simulink model "orbit_propagator_matlab2023b"  (R2023b)
settings: Solver=FixedStepAuto  StartTime=0.0  StopTime=207944  FixedStep=sim_step_size  RelTol=1e-6  AbsTol=1e-7
model workspace (MAT data in the model file):
  current_year = 2025
  year = 2013
values from neighbouring files (symbols this model uses):
  alpha_acc = sqrt(0.7)    [HSat_op_setup_merged_maria.m]    (also in init_orbit_analysis_with_drag_loss.m)
  aph = 200*ones(1,7)    [init_orbit_analysis_with_drag_loss.m]
  COM = [0, 0, 0.25+0.3]    [init_orbit_analysis_with_drag_loss.m]
  ext_ENV_muEarth = 3.986005e14    (= 398600500000000)    [GEO_insertion_setup.m]    (also in HSat_op_setup.m; HSat_op_setup_merged_maria.m; init_orbit_analysis_with_drag_loss.m)
  F107 = 300    [init_orbit_analysis_with_drag_loss.m]
  P_solar = 4.56e-6    (= 4.56e-06)    [HSat_op_setup_merged_maria.m]    (also in init_orbit_analysis_with_drag_loss.m)
  perigee_vector_eci = [0, 1, 0]    [init_orbit_analysis_with_drag_loss.m]
  sim_SC_init_MoI_EOR_wet = [ ... (first row only)    [HSat_op_setup.m]    (also in HSat_op_setup_merged_maria.m; init_orbit_analysis_with_drag_loss.m)
  sim_step_size = 10    [init_orbit_analysis_with_drag_loss.m]
  sun_pointing = 1    [init_orbit_analysis_with_drag_loss.m]
  sun_pointing_SA = 0    [HSat_op_setup_merged_maria.m]    (also in init_orbit_analysis_with_drag_loss.m)
  theta = deg2rad(0)    [init_orbit_analysis_with_drag_loss.m]
undefined symbols (not defined in the file or in its folder): attitude, sun_vector_oc
libraries: aerolibutil x37, matrix_library x37, Toolbox x10, sharedtransform x10, aerolibatmos2 x1, simulink x1, simulink_extras x1
(part 3 of 3)

== system orbit_propagator_matlab2023b/Disturbing torques/sc area projected to v // aero drag torque // srp torque/Switch Case Action Subsystem/sun pointing solar arrays/Nomalize_noDivideByZero1 ==
  e : Inport
  2-norm : Subsystem
      mask Display: disp('||u||')
  Product : Product  Inputs=*/  InputSameDT=on  RndMeth=Zero  SaturateOnIntegerOverflow=on  OutDataTypeStr=Inherit: Same as first input
  Switch : Switch  Criteria=u2 > Threshold  SaturateOnIntegerOverflow=off  InputSameDT=off
  zero : Constant  Value=0
  ehat : Outport
  wires:
  e/1 -> 2-norm/1(In1), Product/1
  2-norm/1(Out1) -> Switch/2, Product/2
  Switch/1 -> ehat/1
  Product/1 -> Switch/1
  zero/1 -> Switch/3

== system orbit_propagator_matlab2023b/Disturbing torques/sc area projected to v // aero drag torque // srp torque/z -1/Nomalize_noDivideByZero/2-norm ==
  In1 : Inport
  Math Function : Math  Operator=sqrt  SignedPower=on
  Product1 : Product  InputSameDT=on  RndMeth=Zero  SaturateOnIntegerOverflow=on  OutDataTypeStr=Inherit: Same as first input
  Sum : Sum  Inputs=+  InputSameDT=on  SaturateOnIntegerOverflow=on  OutDataTypeStr=Inherit: Same as first input
  Out1 : Outport
  wires:
  In1/1 -> Product1/1, Product1/2
  Product1/1 -> Sum/1
  Sum/1 -> Math Function/1
  Math Function/1 -> Out1/1

== system orbit_propagator_matlab2023b/Disturbing torques/sc area projected to v // aero drag torque // srp torque/z -1/Nomalize_noDivideByZero1/2-norm ==
  In1 : Inport
  Math Function : Math  Operator=sqrt  SignedPower=on
  Product1 : Product  InputSameDT=on  RndMeth=Zero  SaturateOnIntegerOverflow=on  OutDataTypeStr=Inherit: Same as first input
  Sum : Sum  Inputs=+  InputSameDT=on  SaturateOnIntegerOverflow=on  OutDataTypeStr=Inherit: Same as first input
  Out1 : Outport
  wires:
  In1/1 -> Product1/1, Product1/2
  Product1/1 -> Sum/1
  Sum/1 -> Math Function/1
  Math Function/1 -> Out1/1

== system orbit_propagator_matlab2023b/Disturbing torques/sc area projected to v // aero drag torque // srp torque/z -2/Nomalize_noDivideByZero/2-norm ==
  In1 : Inport
  Math Function : Math  Operator=sqrt  SignedPower=on
  Product1 : Product  InputSameDT=on  RndMeth=Zero  SaturateOnIntegerOverflow=on  OutDataTypeStr=Inherit: Same as first input
  Sum : Sum  Inputs=+  InputSameDT=on  SaturateOnIntegerOverflow=on  OutDataTypeStr=Inherit: Same as first input
  Out1 : Outport
  wires:
  In1/1 -> Product1/1, Product1/2
  Product1/1 -> Sum/1
  Sum/1 -> Math Function/1
  Math Function/1 -> Out1/1

== system orbit_propagator_matlab2023b/Disturbing torques/sc area projected to v // aero drag torque // srp torque/z -2/Nomalize_noDivideByZero1/2-norm ==
  In1 : Inport
  Math Function : Math  Operator=sqrt  SignedPower=on
  Product1 : Product  InputSameDT=on  RndMeth=Zero  SaturateOnIntegerOverflow=on  OutDataTypeStr=Inherit: Same as first input
  Sum : Sum  Inputs=+  InputSameDT=on  SaturateOnIntegerOverflow=on  OutDataTypeStr=Inherit: Same as first input
  Out1 : Outport
  wires:
  In1/1 -> Product1/1, Product1/2
  Product1/1 -> Sum/1
  Sum/1 -> Math Function/1
  Math Function/1 -> Out1/1

== system orbit_propagator_matlab2023b/Disturbing torques/sc area projected to v // aero drag torque // srp torque/z -3/Nomalize_noDivideByZero/2-norm ==
  In1 : Inport
  Math Function : Math  Operator=sqrt  SignedPower=on
  Product1 : Product  InputSameDT=on  RndMeth=Zero  SaturateOnIntegerOverflow=on  OutDataTypeStr=Inherit: Same as first input
  Sum : Sum  Inputs=+  InputSameDT=on  SaturateOnIntegerOverflow=on  OutDataTypeStr=Inherit: Same as first input
  Out1 : Outport
  wires:
  In1/1 -> Product1/1, Product1/2
  Product1/1 -> Sum/1
  Sum/1 -> Math Function/1
  Math Function/1 -> Out1/1

== system orbit_propagator_matlab2023b/Disturbing torques/sc area projected to v // aero drag torque // srp torque/z -3/Nomalize_noDivideByZero1/2-norm ==
  In1 : Inport
  Math Function : Math  Operator=sqrt  SignedPower=on
  Product1 : Product  InputSameDT=on  RndMeth=Zero  SaturateOnIntegerOverflow=on  OutDataTypeStr=Inherit: Same as first input
  Sum : Sum  Inputs=+  InputSameDT=on  SaturateOnIntegerOverflow=on  OutDataTypeStr=Inherit: Same as first input
  Out1 : Outport
  wires:
  In1/1 -> Product1/1, Product1/2
  Product1/1 -> Sum/1
  Sum/1 -> Math Function/1
  Math Function/1 -> Out1/1

== system orbit_propagator_matlab2023b/Disturbing torques/sc area projected to v // aero drag torque // srp torque/z -4/Nomalize_noDivideByZero/2-norm ==
  In1 : Inport
  Math Function : Math  Operator=sqrt  SignedPower=on
  Product1 : Product  InputSameDT=on  RndMeth=Zero  SaturateOnIntegerOverflow=on  OutDataTypeStr=Inherit: Same as first input
  Sum : Sum  Inputs=+  InputSameDT=on  SaturateOnIntegerOverflow=on  OutDataTypeStr=Inherit: Same as first input
  Out1 : Outport
  wires:
  In1/1 -> Product1/1, Product1/2
  Product1/1 -> Sum/1
  Sum/1 -> Math Function/1
  Math Function/1 -> Out1/1

== system orbit_propagator_matlab2023b/Disturbing torques/sc area projected to v // aero drag torque // srp torque/z -4/Nomalize_noDivideByZero1/2-norm ==
  In1 : Inport
  Math Function : Math  Operator=sqrt  SignedPower=on
  Product1 : Product  InputSameDT=on  RndMeth=Zero  SaturateOnIntegerOverflow=on  OutDataTypeStr=Inherit: Same as first input
  Sum : Sum  Inputs=+  InputSameDT=on  SaturateOnIntegerOverflow=on  OutDataTypeStr=Inherit: Same as first input
  Out1 : Outport
  wires:
  In1/1 -> Product1/1, Product1/2
  Product1/1 -> Sum/1
  Sum/1 -> Math Function/1
  Math Function/1 -> Out1/1

== system orbit_propagator_matlab2023b/Disturbing torques/sc area projected to v // aero drag torque // srp torque/z -5/Nomalize_noDivideByZero/2-norm ==
  In1 : Inport
  Math Function : Math  Operator=sqrt  SignedPower=on
  Product1 : Product  InputSameDT=on  RndMeth=Zero  SaturateOnIntegerOverflow=on  OutDataTypeStr=Inherit: Same as first input
  Sum : Sum  Inputs=+  InputSameDT=on  SaturateOnIntegerOverflow=on  OutDataTypeStr=Inherit: Same as first input
  Out1 : Outport
  wires:
  In1/1 -> Product1/1, Product1/2
  Product1/1 -> Sum/1
  Sum/1 -> Math Function/1
  Math Function/1 -> Out1/1

== system orbit_propagator_matlab2023b/Disturbing torques/sc area projected to v // aero drag torque // srp torque/z -5/Nomalize_noDivideByZero1/2-norm ==
  In1 : Inport
  Math Function : Math  Operator=sqrt  SignedPower=on
  Product1 : Product  InputSameDT=on  RndMeth=Zero  SaturateOnIntegerOverflow=on  OutDataTypeStr=Inherit: Same as first input
  Sum : Sum  Inputs=+  InputSameDT=on  SaturateOnIntegerOverflow=on  OutDataTypeStr=Inherit: Same as first input
  Out1 : Outport
  wires:
  In1/1 -> Product1/1, Product1/2
  Product1/1 -> Sum/1
  Sum/1 -> Math Function/1
  Math Function/1 -> Out1/1

== system orbit_propagator_matlab2023b/Disturbing torques/sc area projected to v // aero drag torque // srp torque/z -6/Nomalize_noDivideByZero/2-norm ==
  In1 : Inport
  Math Function : Math  Operator=sqrt  SignedPower=on
  Product1 : Product  InputSameDT=on  RndMeth=Zero  SaturateOnIntegerOverflow=on  OutDataTypeStr=Inherit: Same as first input
  Sum : Sum  Inputs=+  InputSameDT=on  SaturateOnIntegerOverflow=on  OutDataTypeStr=Inherit: Same as first input
  Out1 : Outport
  wires:
  In1/1 -> Product1/1, Product1/2
  Product1/1 -> Sum/1
  Sum/1 -> Math Function/1
  Math Function/1 -> Out1/1

== system orbit_propagator_matlab2023b/Disturbing torques/sc area projected to v // aero drag torque // srp torque/z -6/Nomalize_noDivideByZero1/2-norm ==
  In1 : Inport
  Math Function : Math  Operator=sqrt  SignedPower=on
  Product1 : Product  InputSameDT=on  RndMeth=Zero  SaturateOnIntegerOverflow=on  OutDataTypeStr=Inherit: Same as first input
  Sum : Sum  Inputs=+  InputSameDT=on  SaturateOnIntegerOverflow=on  OutDataTypeStr=Inherit: Same as first input
  Out1 : Outport
  wires:
  In1/1 -> Product1/1, Product1/2
  Product1/1 -> Sum/1
  Sum/1 -> Math Function/1
  Math Function/1 -> Out1/1

== system orbit_propagator_matlab2023b/Disturbing torques/sc area projected to v // aero drag torque // srp torque/z -7/Nomalize_noDivideByZero/2-norm ==
  In1 : Inport
  Math Function : Math  Operator=sqrt  SignedPower=on
  Product1 : Product  InputSameDT=on  RndMeth=Zero  SaturateOnIntegerOverflow=on  OutDataTypeStr=Inherit: Same as first input
  Sum : Sum  Inputs=+  InputSameDT=on  SaturateOnIntegerOverflow=on  OutDataTypeStr=Inherit: Same as first input
  Out1 : Outport
  wires:
  In1/1 -> Product1/1, Product1/2
  Product1/1 -> Sum/1
  Sum/1 -> Math Function/1
  Math Function/1 -> Out1/1

== system orbit_propagator_matlab2023b/Disturbing torques/sc area projected to v // aero drag torque // srp torque/z -7/Nomalize_noDivideByZero1/2-norm ==
  In1 : Inport
  Math Function : Math  Operator=sqrt  SignedPower=on
  Product1 : Product  InputSameDT=on  RndMeth=Zero  SaturateOnIntegerOverflow=on  OutDataTypeStr=Inherit: Same as first input
  Sum : Sum  Inputs=+  InputSameDT=on  SaturateOnIntegerOverflow=on  OutDataTypeStr=Inherit: Same as first input
  Out1 : Outport
  wires:
  In1/1 -> Product1/1, Product1/2
  Product1/1 -> Sum/1
  Sum/1 -> Math Function/1
  Math Function/1 -> Out1/1

== system orbit_propagator_matlab2023b/Subsystem/Attitude/Att z towards the sun/Nomalize_noDivideByZero1/2-norm ==
  In1 : Inport
  Math Function : Math  Operator=sqrt  SignedPower=on
  Product1 : Product  InputSameDT=on  RndMeth=Zero  SaturateOnIntegerOverflow=on  OutDataTypeStr=Inherit: Same as first input
  Sum : Sum  Inputs=+  InputSameDT=on  SaturateOnIntegerOverflow=on  OutDataTypeStr=Inherit: Same as first input
  Out1 : Outport
  wires:
  In1/1 -> Product1/1, Product1/2
  Product1/1 -> Sum/1
  Sum/1 -> Math Function/1
  Math Function/1 -> Out1/1

== system orbit_propagator_matlab2023b/Subsystem/Attitude/Att z towards the sun/Nomalize_noDivideByZero2/2-norm ==
  In1 : Inport
  Math Function : Math  Operator=sqrt  SignedPower=on
  Product1 : Product  InputSameDT=on  RndMeth=Zero  SaturateOnIntegerOverflow=on  OutDataTypeStr=Inherit: Same as first input
  Sum : Sum  Inputs=+  InputSameDT=on  SaturateOnIntegerOverflow=on  OutDataTypeStr=Inherit: Same as first input
  Out1 : Outport
  wires:
  In1/1 -> Product1/1, Product1/2
  Product1/1 -> Sum/1
  Sum/1 -> Math Function/1
  Math Function/1 -> Out1/1

== system orbit_propagator_matlab2023b/Subsystem/Attitude/Att z towards the sun/Nomalize_noDivideByZero3/2-norm ==
  In1 : Inport
  Math Function : Math  Operator=sqrt  SignedPower=on
  Product1 : Product  InputSameDT=on  RndMeth=Zero  SaturateOnIntegerOverflow=on  OutDataTypeStr=Inherit: Same as first input
  Sum : Sum  Inputs=+  InputSameDT=on  SaturateOnIntegerOverflow=on  OutDataTypeStr=Inherit: Same as first input
  Out1 : Outport
  wires:
  In1/1 -> Product1/1, Product1/2
  Product1/1 -> Sum/1
  Sum/1 -> Math Function/1
  Math Function/1 -> Out1/1

== system orbit_propagator_matlab2023b/Subsystem/Attitude/Att z towards the sun/Nomalize_noDivideByZero4/2-norm ==
  In1 : Inport
  Math Function : Math  Operator=sqrt  SignedPower=on
  Product1 : Product  InputSameDT=on  RndMeth=Zero  SaturateOnIntegerOverflow=on  OutDataTypeStr=Inherit: Same as first input
  Sum : Sum  Inputs=+  InputSameDT=on  SaturateOnIntegerOverflow=on  OutDataTypeStr=Inherit: Same as first input
  Out1 : Outport
  wires:
  In1/1 -> Product1/1, Product1/2
  Product1/1 -> Sum/1
  Sum/1 -> Math Function/1
  Math Function/1 -> Out1/1

== system orbit_propagator_matlab2023b/Subsystem/Attitude/Att z towards the sun and rotation around z/Nomalize_noDivideByZero1/2-norm ==
  In1 : Inport
  Math Function : Math  Operator=sqrt  SignedPower=on
  Product1 : Product  InputSameDT=on  RndMeth=Zero  SaturateOnIntegerOverflow=on  OutDataTypeStr=Inherit: Same as first input
  Sum : Sum  Inputs=+  InputSameDT=on  SaturateOnIntegerOverflow=on  OutDataTypeStr=Inherit: Same as first input
  Out1 : Outport
  wires:
  In1/1 -> Product1/1, Product1/2
  Product1/1 -> Sum/1
  Sum/1 -> Math Function/1
  Math Function/1 -> Out1/1

== system orbit_propagator_matlab2023b/Subsystem/Attitude/Att z towards the sun and rotation around z/Nomalize_noDivideByZero2/2-norm ==
  In1 : Inport
  Math Function : Math  Operator=sqrt  SignedPower=on
  Product1 : Product  InputSameDT=on  RndMeth=Zero  SaturateOnIntegerOverflow=on  OutDataTypeStr=Inherit: Same as first input
  Sum : Sum  Inputs=+  InputSameDT=on  SaturateOnIntegerOverflow=on  OutDataTypeStr=Inherit: Same as first input
  Out1 : Outport
  wires:
  In1/1 -> Product1/1, Product1/2
  Product1/1 -> Sum/1
  Sum/1 -> Math Function/1
  Math Function/1 -> Out1/1

== system orbit_propagator_matlab2023b/Subsystem/Attitude/Att z towards the sun and rotation around z/Nomalize_noDivideByZero3/2-norm ==
  In1 : Inport
  Math Function : Math  Operator=sqrt  SignedPower=on
  Product1 : Product  InputSameDT=on  RndMeth=Zero  SaturateOnIntegerOverflow=on  OutDataTypeStr=Inherit: Same as first input
  Sum : Sum  Inputs=+  InputSameDT=on  SaturateOnIntegerOverflow=on  OutDataTypeStr=Inherit: Same as first input
  Out1 : Outport
  wires:
  In1/1 -> Product1/1, Product1/2
  Product1/1 -> Sum/1
  Sum/1 -> Math Function/1
  Math Function/1 -> Out1/1

== system orbit_propagator_matlab2023b/Subsystem/Attitude/Att z towards the sun and rotation around z/Nomalize_noDivideByZero4/2-norm ==
  In1 : Inport
  Math Function : Math  Operator=sqrt  SignedPower=on
  Product1 : Product  InputSameDT=on  RndMeth=Zero  SaturateOnIntegerOverflow=on  OutDataTypeStr=Inherit: Same as first input
  Sum : Sum  Inputs=+  InputSameDT=on  SaturateOnIntegerOverflow=on  OutDataTypeStr=Inherit: Same as first input
  Out1 : Outport
  wires:
  In1/1 -> Product1/1, Product1/2
  Product1/1 -> Sum/1
  Sum/1 -> Math Function/1
  Math Function/1 -> Out1/1

== system orbit_propagator_matlab2023b/Subsystem/Attitude/att: z in v/Nomalize_noDivideByZero/2-norm ==
  In1 : Inport
  Math Function : Math  Operator=sqrt  SignedPower=on
  Product1 : Product  InputSameDT=on  RndMeth=Zero  SaturateOnIntegerOverflow=on  OutDataTypeStr=Inherit: Same as first input
  Sum : Sum  Inputs=+  InputSameDT=on  SaturateOnIntegerOverflow=on  OutDataTypeStr=Inherit: Same as first input
  Out1 : Outport
  wires:
  In1/1 -> Product1/1, Product1/2
  Product1/1 -> Sum/1
  Sum/1 -> Math Function/1
  Math Function/1 -> Out1/1

== system orbit_propagator_matlab2023b/Subsystem/Attitude/att: z in v/Nomalize_noDivideByZero2/2-norm ==
  In1 : Inport
  Math Function : Math  Operator=sqrt  SignedPower=on
  Product1 : Product  InputSameDT=on  RndMeth=Zero  SaturateOnIntegerOverflow=on  OutDataTypeStr=Inherit: Same as first input
  Sum : Sum  Inputs=+  InputSameDT=on  SaturateOnIntegerOverflow=on  OutDataTypeStr=Inherit: Same as first input
  Out1 : Outport
  wires:
  In1/1 -> Product1/1, Product1/2
  Product1/1 -> Sum/1
  Sum/1 -> Math Function/1
  Math Function/1 -> Out1/1

== system orbit_propagator_matlab2023b/Subsystem/Attitude/att: z in v/Nomalize_noDivideByZero4/2-norm ==
  In1 : Inport
  Math Function : Math  Operator=sqrt  SignedPower=on
  Product1 : Product  InputSameDT=on  RndMeth=Zero  SaturateOnIntegerOverflow=on  OutDataTypeStr=Inherit: Same as first input
  Sum : Sum  Inputs=+  InputSameDT=on  SaturateOnIntegerOverflow=on  OutDataTypeStr=Inherit: Same as first input
  Out1 : Outport
  wires:
  In1/1 -> Product1/1, Product1/2
  Product1/1 -> Sum/1
  Sum/1 -> Math Function/1
  Math Function/1 -> Out1/1

== system orbit_propagator_matlab2023b/Subsystem/Attitude/changes with altitude/q (x in v)/Nomalize_noDivideByZero ==
  e : Inport
  2-norm : Subsystem
      mask Display: disp('||u||')
  Product : Product  Inputs=*/  InputSameDT=on  RndMeth=Zero  SaturateOnIntegerOverflow=on  OutDataTypeStr=Inherit: Same as first input
  Switch : Switch  Criteria=u2 > Threshold  SaturateOnIntegerOverflow=off  InputSameDT=off
  zero : Constant  Value=0
  ehat : Outport
  wires:
  e/1 -> 2-norm/1(In1), Product/1
  2-norm/1(Out1) -> Switch/2, Product/2
  Switch/1 -> ehat/1
  Product/1 -> Switch/1
  zero/1 -> Switch/3

== system orbit_propagator_matlab2023b/Subsystem/Attitude/changes with altitude/q (x in v)/Nomalize_noDivideByZero1 ==
  e : Inport
  2-norm : Subsystem
      mask Display: disp('||u||')
  Product : Product  Inputs=*/  InputSameDT=on  RndMeth=Zero  SaturateOnIntegerOverflow=on  OutDataTypeStr=Inherit: Same as first input
  Switch : Switch  Criteria=u2 > Threshold  SaturateOnIntegerOverflow=off  InputSameDT=off
  zero : Constant  Value=0
  ehat : Outport
  wires:
  e/1 -> 2-norm/1(In1), Product/1
  2-norm/1(Out1) -> Switch/2, Product/2
  Switch/1 -> ehat/1
  Product/1 -> Switch/1
  zero/1 -> Switch/3

== system orbit_propagator_matlab2023b/Subsystem/Attitude/changes with altitude/q (x in v)/Nomalize_noDivideByZero2 ==
  e : Inport
  2-norm : Subsystem
      mask Display: disp('||u||')
  Product : Product  Inputs=*/  InputSameDT=on  RndMeth=Zero  SaturateOnIntegerOverflow=on  OutDataTypeStr=Inherit: Same as first input
  Switch : Switch  Criteria=u2 > Threshold  SaturateOnIntegerOverflow=off  InputSameDT=off
  zero : Constant  Value=0
  ehat : Outport
  wires:
  e/1 -> 2-norm/1(In1), Product/1
  2-norm/1(Out1) -> Switch/2, Product/2
  Switch/1 -> ehat/1
  Product/1 -> Switch/1
  zero/1 -> Switch/3

== system orbit_propagator_matlab2023b/Subsystem/Attitude/changes with altitude/q (x in v)/Nomalize_noDivideByZero4 ==
  e : Inport
  2-norm : Subsystem
      mask Display: disp('||u||')
  Product : Product  Inputs=*/  InputSameDT=on  RndMeth=Zero  SaturateOnIntegerOverflow=on  OutDataTypeStr=Inherit: Same as first input
  Switch : Switch  Criteria=u2 > Threshold  SaturateOnIntegerOverflow=off  InputSameDT=off
  zero : Constant  Value=0
  ehat : Outport
  wires:
  e/1 -> 2-norm/1(In1), Product/1
  2-norm/1(Out1) -> Switch/2, Product/2
  Switch/1 -> ehat/1
  Product/1 -> Switch/1
  zero/1 -> Switch/3

== system orbit_propagator_matlab2023b/Subsystem/Attitude/changes with altitude/q (z in r)/Nomalize_noDivideByZero ==
  e : Inport
  2-norm : Subsystem
      mask Display: disp('||u||')
  Product : Product  Inputs=*/  InputSameDT=on  RndMeth=Zero  SaturateOnIntegerOverflow=on  OutDataTypeStr=Inherit: Same as first input
  Switch : Switch  Criteria=u2 > Threshold  SaturateOnIntegerOverflow=off  InputSameDT=off
  zero : Constant  Value=0
  ehat : Outport
  wires:
  e/1 -> 2-norm/1(In1), Product/1
  2-norm/1(Out1) -> Switch/2, Product/2
  Switch/1 -> ehat/1
  Product/1 -> Switch/1
  zero/1 -> Switch/3

== system orbit_propagator_matlab2023b/Subsystem/Attitude/changes with altitude/q (z in r)/Nomalize_noDivideByZero2 ==
  e : Inport
  2-norm : Subsystem
      mask Display: disp('||u||')
  Product : Product  Inputs=*/  InputSameDT=on  RndMeth=Zero  SaturateOnIntegerOverflow=on  OutDataTypeStr=Inherit: Same as first input
  Switch : Switch  Criteria=u2 > Threshold  SaturateOnIntegerOverflow=off  InputSameDT=off
  zero : Constant  Value=0
  ehat : Outport
  wires:
  e/1 -> 2-norm/1(In1), Product/1
  2-norm/1(Out1) -> Switch/2, Product/2
  Switch/1 -> ehat/1
  Product/1 -> Switch/1
  zero/1 -> Switch/3

== system orbit_propagator_matlab2023b/Subsystem/Attitude/changes with altitude/q (z in r)/Nomalize_noDivideByZero4 ==
  e : Inport
  2-norm : Subsystem
      mask Display: disp('||u||')
  Product : Product  Inputs=*/  InputSameDT=on  RndMeth=Zero  SaturateOnIntegerOverflow=on  OutDataTypeStr=Inherit: Same as first input
  Switch : Switch  Criteria=u2 > Threshold  SaturateOnIntegerOverflow=off  InputSameDT=off
  zero : Constant  Value=0
  ehat : Outport
  wires:
  e/1 -> 2-norm/1(In1), Product/1
  2-norm/1(Out1) -> Switch/2, Product/2
  Switch/1 -> ehat/1
  Product/1 -> Switch/1
  zero/1 -> Switch/3

== system orbit_propagator_matlab2023b/Subsystem/Attitude/changes with altitude/q (z in v)/Nomalize_noDivideByZero ==
  e : Inport
  2-norm : Subsystem
      mask Display: disp('||u||')
  Product : Product  Inputs=*/  InputSameDT=on  RndMeth=Zero  SaturateOnIntegerOverflow=on  OutDataTypeStr=Inherit: Same as first input
  Switch : Switch  Criteria=u2 > Threshold  SaturateOnIntegerOverflow=off  InputSameDT=off
  zero : Constant  Value=0
  ehat : Outport
  wires:
  e/1 -> 2-norm/1(In1), Product/1
  2-norm/1(Out1) -> Switch/2, Product/2
  Switch/1 -> ehat/1
  Product/1 -> Switch/1
  zero/1 -> Switch/3

== system orbit_propagator_matlab2023b/Subsystem/Attitude/changes with altitude/q (z in v)/Nomalize_noDivideByZero2 ==
  e : Inport
  2-norm : Subsystem
      mask Display: disp('||u||')
  Product : Product  Inputs=*/  InputSameDT=on  RndMeth=Zero  SaturateOnIntegerOverflow=on  OutDataTypeStr=Inherit: Same as first input
  Switch : Switch  Criteria=u2 > Threshold  SaturateOnIntegerOverflow=off  InputSameDT=off
  zero : Constant  Value=0
  ehat : Outport
  wires:
  e/1 -> 2-norm/1(In1), Product/1
  2-norm/1(Out1) -> Switch/2, Product/2
  Switch/1 -> ehat/1
  Product/1 -> Switch/1
  zero/1 -> Switch/3

== system orbit_propagator_matlab2023b/Subsystem/Attitude/changes with altitude/q (z in v)/Nomalize_noDivideByZero4 ==
  e : Inport
  2-norm : Subsystem
      mask Display: disp('||u||')
  Product : Product  Inputs=*/  InputSameDT=on  RndMeth=Zero  SaturateOnIntegerOverflow=on  OutDataTypeStr=Inherit: Same as first input
  Switch : Switch  Criteria=u2 > Threshold  SaturateOnIntegerOverflow=off  InputSameDT=off
  zero : Constant  Value=0
  ehat : Outport
  wires:
  e/1 -> 2-norm/1(In1), Product/1
  2-norm/1(Out1) -> Switch/2, Product/2
  Switch/1 -> ehat/1
  Product/1 -> Switch/1
  zero/1 -> Switch/3

== system orbit_propagator_matlab2023b/Subsystem/Attitude/q (z in r)/Nomalize_noDivideByZero/2-norm ==
  In1 : Inport
  Math Function : Math  Operator=sqrt  SignedPower=on
  Product1 : Product  InputSameDT=on  RndMeth=Zero  SaturateOnIntegerOverflow=on  OutDataTypeStr=Inherit: Same as first input
  Sum : Sum  Inputs=+  InputSameDT=on  SaturateOnIntegerOverflow=on  OutDataTypeStr=Inherit: Same as first input
  Out1 : Outport
  wires:
  In1/1 -> Product1/1, Product1/2
  Product1/1 -> Sum/1
  Sum/1 -> Math Function/1
  Math Function/1 -> Out1/1

== system orbit_propagator_matlab2023b/Subsystem/Attitude/q (z in r)/Nomalize_noDivideByZero2/2-norm ==
  In1 : Inport
  Math Function : Math  Operator=sqrt  SignedPower=on
  Product1 : Product  InputSameDT=on  RndMeth=Zero  SaturateOnIntegerOverflow=on  OutDataTypeStr=Inherit: Same as first input
  Sum : Sum  Inputs=+  InputSameDT=on  SaturateOnIntegerOverflow=on  OutDataTypeStr=Inherit: Same as first input
  Out1 : Outport
  wires:
  In1/1 -> Product1/1, Product1/2
  Product1/1 -> Sum/1
  Sum/1 -> Math Function/1
  Math Function/1 -> Out1/1

== system orbit_propagator_matlab2023b/Subsystem/Attitude/q (z in r)/Nomalize_noDivideByZero4/2-norm ==
  In1 : Inport
  Math Function : Math  Operator=sqrt  SignedPower=on
  Product1 : Product  InputSameDT=on  RndMeth=Zero  SaturateOnIntegerOverflow=on  OutDataTypeStr=Inherit: Same as first input
  Sum : Sum  Inputs=+  InputSameDT=on  SaturateOnIntegerOverflow=on  OutDataTypeStr=Inherit: Same as first input
  Out1 : Outport
  wires:
  In1/1 -> Product1/1, Product1/2
  Product1/1 -> Sum/1
  Sum/1 -> Math Function/1
  Math Function/1 -> Out1/1

== system orbit_propagator_matlab2023b/Disturbing torques/sc area projected to v // aero drag torque // srp torque/Switch Case Action Subsystem/sun pointing solar arrays/Nomalize_noDivideByZero1/2-norm ==
  In1 : Inport
  Math Function : Math  Operator=sqrt  SignedPower=on
  Product1 : Product  InputSameDT=on  RndMeth=Zero  SaturateOnIntegerOverflow=on  OutDataTypeStr=Inherit: Same as first input
  Sum : Sum  Inputs=+  InputSameDT=on  SaturateOnIntegerOverflow=on  OutDataTypeStr=Inherit: Same as first input
  Out1 : Outport
  wires:
  In1/1 -> Product1/1, Product1/2
  Product1/1 -> Sum/1
  Sum/1 -> Math Function/1
  Math Function/1 -> Out1/1

== system orbit_propagator_matlab2023b/Subsystem/Attitude/changes with altitude/q (x in v)/Nomalize_noDivideByZero/2-norm ==
  In1 : Inport
  Math Function : Math  Operator=sqrt  SignedPower=on
  Product1 : Product  InputSameDT=on  RndMeth=Zero  SaturateOnIntegerOverflow=on  OutDataTypeStr=Inherit: Same as first input
  Sum : Sum  Inputs=+  InputSameDT=on  SaturateOnIntegerOverflow=on  OutDataTypeStr=Inherit: Same as first input
  Out1 : Outport
  wires:
  In1/1 -> Product1/1, Product1/2
  Product1/1 -> Sum/1
  Sum/1 -> Math Function/1
  Math Function/1 -> Out1/1

== system orbit_propagator_matlab2023b/Subsystem/Attitude/changes with altitude/q (x in v)/Nomalize_noDivideByZero1/2-norm ==
  In1 : Inport
  Math Function : Math  Operator=sqrt  SignedPower=on
  Product1 : Product  InputSameDT=on  RndMeth=Zero  SaturateOnIntegerOverflow=on  OutDataTypeStr=Inherit: Same as first input
  Sum : Sum  Inputs=+  InputSameDT=on  SaturateOnIntegerOverflow=on  OutDataTypeStr=Inherit: Same as first input
  Out1 : Outport
  wires:
  In1/1 -> Product1/1, Product1/2
  Product1/1 -> Sum/1
  Sum/1 -> Math Function/1
  Math Function/1 -> Out1/1

== system orbit_propagator_matlab2023b/Subsystem/Attitude/changes with altitude/q (x in v)/Nomalize_noDivideByZero2/2-norm ==
  In1 : Inport
  Math Function : Math  Operator=sqrt  SignedPower=on
  Product1 : Product  InputSameDT=on  RndMeth=Zero  SaturateOnIntegerOverflow=on  OutDataTypeStr=Inherit: Same as first input
  Sum : Sum  Inputs=+  InputSameDT=on  SaturateOnIntegerOverflow=on  OutDataTypeStr=Inherit: Same as first input
  Out1 : Outport
  wires:
  In1/1 -> Product1/1, Product1/2
  Product1/1 -> Sum/1
  Sum/1 -> Math Function/1
  Math Function/1 -> Out1/1

== system orbit_propagator_matlab2023b/Subsystem/Attitude/changes with altitude/q (x in v)/Nomalize_noDivideByZero4/2-norm ==
  In1 : Inport
  Math Function : Math  Operator=sqrt  SignedPower=on
  Product1 : Product  InputSameDT=on  RndMeth=Zero  SaturateOnIntegerOverflow=on  OutDataTypeStr=Inherit: Same as first input
  Sum : Sum  Inputs=+  InputSameDT=on  SaturateOnIntegerOverflow=on  OutDataTypeStr=Inherit: Same as first input
  Out1 : Outport
  wires:
  In1/1 -> Product1/1, Product1/2
  Product1/1 -> Sum/1
  Sum/1 -> Math Function/1
  Math Function/1 -> Out1/1

== system orbit_propagator_matlab2023b/Subsystem/Attitude/changes with altitude/q (z in r)/Nomalize_noDivideByZero/2-norm ==
  In1 : Inport
  Math Function : Math  Operator=sqrt  SignedPower=on
  Product1 : Product  InputSameDT=on  RndMeth=Zero  SaturateOnIntegerOverflow=on  OutDataTypeStr=Inherit: Same as first input
  Sum : Sum  Inputs=+  InputSameDT=on  SaturateOnIntegerOverflow=on  OutDataTypeStr=Inherit: Same as first input
  Out1 : Outport
  wires:
  In1/1 -> Product1/1, Product1/2
  Product1/1 -> Sum/1
  Sum/1 -> Math Function/1
  Math Function/1 -> Out1/1

== system orbit_propagator_matlab2023b/Subsystem/Attitude/changes with altitude/q (z in r)/Nomalize_noDivideByZero2/2-norm ==
  In1 : Inport
  Math Function : Math  Operator=sqrt  SignedPower=on
  Product1 : Product  InputSameDT=on  RndMeth=Zero  SaturateOnIntegerOverflow=on  OutDataTypeStr=Inherit: Same as first input
  Sum : Sum  Inputs=+  InputSameDT=on  SaturateOnIntegerOverflow=on  OutDataTypeStr=Inherit: Same as first input
  Out1 : Outport
  wires:
  In1/1 -> Product1/1, Product1/2
  Product1/1 -> Sum/1
  Sum/1 -> Math Function/1
  Math Function/1 -> Out1/1

== system orbit_propagator_matlab2023b/Subsystem/Attitude/changes with altitude/q (z in r)/Nomalize_noDivideByZero4/2-norm ==
  In1 : Inport
  Math Function : Math  Operator=sqrt  SignedPower=on
  Product1 : Product  InputSameDT=on  RndMeth=Zero  SaturateOnIntegerOverflow=on  OutDataTypeStr=Inherit: Same as first input
  Sum : Sum  Inputs=+  InputSameDT=on  SaturateOnIntegerOverflow=on  OutDataTypeStr=Inherit: Same as first input
  Out1 : Outport
  wires:
  In1/1 -> Product1/1, Product1/2
  Product1/1 -> Sum/1
  Sum/1 -> Math Function/1
  Math Function/1 -> Out1/1

== system orbit_propagator_matlab2023b/Subsystem/Attitude/changes with altitude/q (z in v)/Nomalize_noDivideByZero/2-norm ==
  In1 : Inport
  Math Function : Math  Operator=sqrt  SignedPower=on
  Product1 : Product  InputSameDT=on  RndMeth=Zero  SaturateOnIntegerOverflow=on  OutDataTypeStr=Inherit: Same as first input
  Sum : Sum  Inputs=+  InputSameDT=on  SaturateOnIntegerOverflow=on  OutDataTypeStr=Inherit: Same as first input
  Out1 : Outport
  wires:
  In1/1 -> Product1/1, Product1/2
  Product1/1 -> Sum/1
  Sum/1 -> Math Function/1
  Math Function/1 -> Out1/1

== system orbit_propagator_matlab2023b/Subsystem/Attitude/changes with altitude/q (z in v)/Nomalize_noDivideByZero2/2-norm ==
  In1 : Inport
  Math Function : Math  Operator=sqrt  SignedPower=on
  Product1 : Product  InputSameDT=on  RndMeth=Zero  SaturateOnIntegerOverflow=on  OutDataTypeStr=Inherit: Same as first input
  Sum : Sum  Inputs=+  InputSameDT=on  SaturateOnIntegerOverflow=on  OutDataTypeStr=Inherit: Same as first input
  Out1 : Outport
  wires:
  In1/1 -> Product1/1, Product1/2
  Product1/1 -> Sum/1
  Sum/1 -> Math Function/1
  Math Function/1 -> Out1/1

== system orbit_propagator_matlab2023b/Subsystem/Attitude/changes with altitude/q (z in v)/Nomalize_noDivideByZero4/2-norm ==
  In1 : Inport
  Math Function : Math  Operator=sqrt  SignedPower=on
  Product1 : Product  InputSameDT=on  RndMeth=Zero  SaturateOnIntegerOverflow=on  OutDataTypeStr=Inherit: Same as first input
  Sum : Sum  Inputs=+  InputSameDT=on  SaturateOnIntegerOverflow=on  OutDataTypeStr=Inherit: Same as first input
  Out1 : Outport
  wires:
  In1/1 -> Product1/1, Product1/2
  Product1/1 -> Sum/1
  Sum/1 -> Math Function/1
  Math Function/1 -> Out1/1

== matlab function orbit_propagator_matlab2023b/Subsystem/Attitude/Att z towards the sun and rotation around z/MATLAB Function ==
  data: theta input; M output
function M = rot_matrix(theta)

M = [cos(theta), -sin(theta), 0; sin(theta), cos(theta), 0; 0, 0, 1];

== matlab function orbit_propagator_matlab2023b/MATLAB Function ==
  data: r input; coe output; v input
%SV2KEP.M
%
%function kepvec=sv2kep(rsc,vsc)
%
%DESCRIPTION
%Converts from state vector (rvec,vvec) formulation to keplerian elements
%
%INPUT:		rsc	 (3x1) or (3xn) orbit radius vector
%				vsc (3x1) or (3xn) velocity vector
%
%OUTPUT:    	kepvec - (6x1) or (6xn) vector with the keplerian elements
%USES:
%REFERENCE:
%AUTHOR:      	B Jakobsson
%VERSION: 	   92-08-17
%	   	      95-10-02
%				BJA, Sept 2001, vector input accepted, vector output added

% function coe=sv2kep(rvec,vvec)
% 
% if 0
% [p,sma,ecc,incl,an,ap,tran,E,M,arglat,truelon,lonper ] = rv2coe (rvec,vvec);
% coe=[sma ecc incl an ap tran, E, M,arglat,truelon,lonper ]';
% else
%     coe = rv2coe (rvec,vvec);
% end
  
%
% ------------------------------------------------------------------------------
%
%                           function rv2coe
%
%  this function finds the classical orbital elements given the geocentric
%    equatorial position and velocity vectors.
%
%  author        : david vallado                  719-573-2600   21 jun 2002
%
%  revisions
%    vallado     - fix special cases                              5 sep 2002
%    vallado     - delete extra check in inclination code        16 oct 2002
%    vallado     - add constant file use                         29 jun 2003
%    vallado     - add mu                                         2 apr 2007
%
%  inputs          description                    range / units
%    r           - ijk position vector            km
%    v           - ijk velocity vector            km / s
%    mu          - gravitational parameter        km3 / s2
%
%  outputs       :
%    p           - semilatus rectum               km
%    a           - semimajor axis                 km
%    ecc         - eccentricity
%    incl        - inclination                    0.0  to pi rad
%    omega       - longitude of ascending node    0.0  to 2pi rad
%    argp        - argument of perigee            0.0  to 2pi rad
%    nu          - true anomaly                   0.0  to 2pi rad
%    m           - mean anomaly                   0.0  to 2pi rad
%    arglat      - argument of latitude      (ci) 0.0  to 2pi rad
%    truelon     - true longitude            (ce) 0.0  to 2pi rad
%    lonper      - longitude of periapsis    (ee) 0.0  to 2pi rad
%
%  locals        :
%    hbar        - angular momentum h vector      km2 / s
%    ebar        - eccentricity     e vector
%    nbar        - line of nodes    n vector
%    c1          - v**2 - u/r
%    rdotv       - r dot v
%    hk          - hk unit vector
%    sme         - specfic mechanical energy      km2 / s2
%    i           - index
%    e           - eccentric, parabolic,
%                  hyperbolic anomaly             rad
%    temp        - temporary variable
%    typeorbit   - type of orbit                  ee, ei, ce, ci
%
%  coupling      :
%    mag         - magnitude of a vector
%    angl        - find the angl between two vectors
%    newtonnu    - find the mean anomaly
%
%  references    :
%    vallado       2007, 121, alg 9, ex 2-5
%
% [p,a,ecc,incl,omega,argp,nu,m,arglat,truelon,lonper ] = rv2coe (r,v);
% ------------------------------------------------------------------------------

  %  function [p,a,ecc,incl,omega,argp,nu,e,m,arglat,truelon,lonper ] = rv2coe (r,v);
     function coe = rv2coe (r,v)
        
        %  constmath;
        small=1e-10;
        infinite  = 999999.9;
        undefined = 999999.1;
        % -------------------------  mathematical  --------------------
        rad    = 180.0 / pi;
        twopi  = 2.0 * pi;
        halfpi = pi * 0.5;
        
        % constastro;  % don't overwrite mu
        mu=3.986005e14;
        muin = mu; % this is the km version
        % -------------------------  implementation   -----------------
        magr = norm( r );
        magv = norm( v );
        % ------------------  find h n and e vectors   ----------------
        [hbar] = cross( r,v );
        nbar=hbar*NaN;
        ebar=hbar*NaN;
        magh = mag( hbar );
        if ( magh > small )
            nbar(1)= -hbar(2);
            nbar(2)=  hbar(1);
            nbar(3)=   0.0;
            magn = mag( nbar );
            c1 = magv*magv - muin /magr;
            rdotv= dot( r,v );
            for i= 1 : 3
                ebar(i)= (c1*r(i) - rdotv*v(i))/muin;
            end
            ecc = mag( ebar );
            
            % ------------  find a e and semi-latus rectum   ----------
            sme= ( magv*magv*0.5  ) - ( muin /magr );
            if ( abs( sme ) > small )
                a= -muin  / (2.0 *sme);
            else
                a= infinite;
            end
            p = magh*magh/muin;
            
            % -----------------  find inclination   -------------------
            hk= hbar(3)/magh;
            incl= acos( hk );
            
            % --------  determine type of orbit for later use  --------
            % ------ elliptical, parabolic, hyperbolic inclined -------
            typeorbit= 'ei';
            if ( ecc < small )
                % ----------------  circular equatorial ---------------
                if  (incl<small) || (abs(incl-pi)<small)
                    typeorbit= 'ce';
                else
                    % --------------  circular inclined ---------------
                    typeorbit= 'ci';
                end
            else
                % - elliptical, parabolic, hyperbolic equatorial --
                if  (incl<small) || (abs(incl-pi)<small)
                    typeorbit= 'ee';
                end
            end
            
            % ----------  find longitude of ascending node ------------
            if ( magn > small )
                temp= nbar(1) / magn;
                if ( abs(temp) > 1.0  )
                    temp= sign(temp);
                end
                omega= acos( temp );
                if ( nbar(2) < 0.0  )
                    omega= twopi - omega;
                end
            else
                omega= undefined;
            end
            
            % ---------------- find argument of perigee ---------------
            if (strcmp(typeorbit, 'ei') == 1)
                argp = angl( nbar,ebar);
                if ( ebar(3) < 0.0  )
                    argp= twopi - argp;
                end
            else
                argp= undefined;
            end
            
            % ------------  find true anomaly at epoch    -------------
            if ( typeorbit(1:1) == 'e' )
                nu =  angl( ebar,r);
                if ( rdotv < 0.0  )
                    nu= twopi - nu;
                end
            else
                nu= undefined;
            end
            
            % ----  find argument of latitude - circular inclined -----
            if (strcmp(typeorbit, 'ci') == 1)
                arglat = angl( nbar,r );
                if ( r(3) < 0.0  )
                    arglat= twopi - arglat;
                end
                m = arglat;
            else
                arglat= undefined;
            end
            
            % -- find longitude of perigee - elliptical equatorial ----
            if  ( ecc>small ) && (strcmp(typeorbit, 'ee') == 1)
                temp= ebar(1)/ecc;
                if ( abs(temp) > 1.0  )
                    temp= sign(temp);
                end
                lonper= acos( temp );
                if ( ebar(2) < 0.0  )
                    lonper= twopi - lonper;
                end
                if ( incl > halfpi )
                    lonper= twopi - lonper;
                end
            else
                lonper= undefined;
            end
            
            % -------- find true longitude - circular equatorial ------
            if  ( magr>small ) && (strcmp(typeorbit, 'ce') == 1)
                temp= r(1)/magr;
                if ( abs(temp) > 1.0  )
                    temp= sign(temp);
                end
                truelon= acos( temp );
                if ( r(2) < 0.0  )
                    truelon= twopi - truelon;
                end
                if ( incl > halfpi )
                    truelon= twopi - truelon;
                end
                m = truelon;
            else
                truelon= undefined;
            end
            
            % ------------ find mean anomaly for all orbits -----------
            if ( typeorbit(1:1) == 'e' )
                [e,m] = newtonnu(ecc,nu );
            else
                e=undefined;
                m=undefined;
                
            end
            
        else
            p    = undefined;
            a    = undefined;
            ecc  = undefined;
            incl = undefined;
            omega= undefined;
            argp = undefined;
            nu   = undefined;
            m    = undefined;
            e    = undefined;
            arglat = undefined;
            truelon= undefined;
            lonper = undefined;
        end
%coe=[sma ecc incl an ap tran, E, M,arglat,truelon,lonper ]
coe=[  a,ecc,incl,omega,argp,nu,e,m,arglat,truelon,lonper ]';
    end
% end

== matlab function orbit_propagator_matlab2023b/Atmospheric model/MATLAB Function1 ==
  data: julianDate input; yr output; dayOfYear output; timeUTSeconds output
function [yr, dayOfYear, timeUTSeconds] = convertJulianDate(julianDate)
    % Define constants
    secondsInDay = 86400; % Number of seconds in a day
    
    % Calculate year and day of the year
    %J0 = datetime(julianDate, 'convertfrom','juliandate');
    %yr = year(J0);
    [yr, mon, d]= splitymd(jd2ymd(julianDate));

 
    daysInMonth = [31, 28, 31, 30, 31, 30, 31, 31, 30, 31, 30, 31];
    
    % Adjust for leap year
    if mod(yr, 4) == 0 && (mod(yr, 100) ~= 0 || mod(yr, 400) == 0)
        daysInMonth(2) = 29; % February has 29 days in a leap year
    end
   
    
    dayOfYear = sum(daysInMonth(1:mon - 1)) + d;

    
    % Calculate time in UT seconds
    fractionalDay = julianDate - floor(julianDate);
    if fractionalDay < 0.5
        timeUTSeconds = (fractionalDay+0.5) * secondsInDay;
    else
        timeUTSeconds = (fractionalDay-0.5) * secondsInDay;
    end
end
